simulink model "INTEGRATION_TEST_01"  (Simulink 8.1)
settings: Solver=ode4  StartTime=0.0  StopTime=inf  FixedStep=Ts  MaxStep=1e-3  RelTol=1e-3
PostLoadFcn:
  | INTEGRATION_TEST_01_init;
InitFcn:
  | INTEGRATION_TEST_01_init;
values from neighbouring files (symbols this model uses):
  Ts = 100E-6    (= 0.0001)    [INTEGRATION_TEST_01_init.m]
undefined symbols (not defined in the file or in its folder): cable_spec, fdesignblkfcn, gcbh, generic_ethernet_cb, Left, relay_par, type, V
libraries: powerlib_extras x14, rtio_opalrt_common x13, rtlab x10, cables_lib x6, breaker_lib x4, simulink_extras x4, simulink x4, Load_lib x3, rtio_generic_modbus x3, powerlib x2, ssn_lib x2, transformer_lib x2
(part 2 of 2)

== system INTEGRATION_TEST_01/SS_Relays_and_Woodward/HWCtrl/GR1 B AIN (CH00-15) ==
  AnalogIn : rtio_opalrt_common/AnalogIn  CtrlName='OpCtrl'  portNb=1  FcnNos=Slot 1 Module B Subsection 1  size=16  maxcount=8  count=8  numchan=8  sampleTime=0
      settings: AttributesFormatString=%<CtrlName>
  AnalogIn1 : rtio_opalrt_common/AnalogIn  CtrlName='OpCtrl'  portNb=2  FcnNos=Slot 1 Module B Subsection 2  size=16  maxcount=8  count=8  numchan=8  sampleTime=0
      settings: AttributesFormatString=%<CtrlName>
  Mux6 : Mux  Inputs=2
  Terminator2 : Terminator
  Terminator3 : Terminator
  Out1 : Outport
  wires:
  AnalogIn/1 -> Mux6/1
  AnalogIn1/1 -> Mux6/2
  AnalogIn/2 -> Terminator2/1
  AnalogIn1/2 -> Terminator3/1
  Mux6/1 -> Out1/1

== system INTEGRATION_TEST_01/SS_Relays_and_Woodward/HWCtrl/SEL751_DigitalAnalog_IO_OpBlocks ==
  note: This connector also services Genset #2 and  is
      | shared with Genset #1.  Use RJ45 connectors to
      |  intercept Genset #2 I/O (not used in this Device
      | Integration Test) and use for SEL-751
  note: Remove existing connections to Slot 3 I/O, if any
      | ans replace with connections shown below, or use
      | corresponding RJ45 connectors.  (Existing I/O, if any not
      |  used for this Device Integration Test)
  note: When the system uses the simulated
      | Secondary Controller the digital I/O
      | should be disabled.
  note: Copyright (c) 2016 Massachusetts Institute of Technology
      | Permission is hereby granted, free of charge, to any person obtaining a copy of this software and associated documentation files (the "Software"), to deal
      | in the Software without restriction, including without limitation the rights to use, copy, modify, merge, publish, distribute, sublicense, and/or sell copies of the
      | Software, and to permit persons to whom the Software is furnished to do so, subject to the following conditions:
      |
      | THE SOFTWARE IS PROVIDED "AS IS", WITHOUT WARRANTY OF ANY KIND, EXPRESS OR IMPLIED, INCLUDING BUT NOT LIMITED TO THE
      | WARRANTIES OF MERCHANTABILITY, FITNESS FOR A PARTICULAR PURPOSE AND NONINFRINGEMENT. IN NO EVENT SHALL THE AUTHORS
      | OR COPYRIGHT HOLDERS BE LIABLE FOR ANY CLAIM, DAMAGES OR OTHER LIABILITY, WHETHER IN AN ACTION OF CONTRACT, TORT OR
      | OTHERWISE, ARISING FROM, OUT OF OR IN CONNECTION WITH THE SOFTWARE OR THE USE OR OTHER DEALINGS IN THE SOFTWARE
  SEL751-01_ScaledSignals : Inport
  AnalogOut2 to SEL-751 : rtio_opalrt_common/AnalogOut  CtrlName='OpCtrl'  portNb=4  FcnNos=Slot 2 Module A Subsection 2  size=16  maxcount=8  count=8  numchan=8  israngeinput=off  voltagerange=[ -5 ... 5 ]  slot=1  side=0  mismatch=0  slotside=Slot_2_Module_A
      settings: AttributesFormatString=%<CtrlName>
  Bus Creator4 : BusCreator  Inputs=2
  Bus Selector4 : BusSelector  OutputSignals=To DigitalOut_to_SEL-751,To AnalogOut_to_SEL-751
  Data Type Conversion{,1..3} (4 alike) : DataTypeConversion
  Demux6 : Demux  Outputs=8
  DigitalIn from SEL-751 : rtio_opalrt_common/DigitalIn  CtrlName='OpCtrl'  portNb=6  FcnNos=Slot 3 Module A Subsection 2  size=1  maxcount=8  count=8  sampleTime=Ts  numchan=8
      settings: AttributesFormatString=%<CtrlName>
  DigitalOut to SEL-751 : rtio_opalrt_common/DigitalOut  CtrlName='OpCtrl'  portNb=6  FcnNos=Slot 3 Module B Subsection 2  size=1  maxcount=8  count=8  numchan=8
      settings: AttributesFormatString=%<CtrlName>
  S-R Flip-Flop : simulink_extras/Flip Flops/S-R Flip-Flop  initial_condition=1
  Terminator : Terminator
  Terminator1 : Terminator
  Terminator2 : Terminator
  SEL751-01_LogicTrip : Outport
  wires:
  DigitalOut to SEL-751/1 -> Terminator1/1
  AnalogOut2 to SEL-751/1 -> Terminator/1
  Demux6/2 -> Data Type Conversion1/1  "OUT102 Brkr reset"
  Demux6/1 -> Data Type Conversion/1  "OUT103 Brkr trip"
  Data Type Conversion3/1 -> Bus Creator4/2  "Logic_reset"
  Data Type Conversion/1 -> S-R Flip-Flop/1
  Bus Selector4/2 -> AnalogOut2 to SEL-751/1  "<To AnalogOut_to_SEL-751>"
  Bus Selector4/1 -> DigitalOut to SEL-751/1  "<To DigitalOut_to_SEL-751>"
  DigitalIn from SEL-751/2 -> Terminator2/1
  SEL751-01_ScaledSignals/1 -> Bus Selector4/1
  DigitalIn from SEL-751/1 -> Demux6/1
  Data Type Conversion1/1 -> S-R Flip-Flop/2
  Data Type Conversion2/1 -> Bus Creator4/1  "Logic_trip"
  Bus Creator4/1 -> SEL751-01_LogicTrip/1
  S-R Flip-Flop/1 -> Data Type Conversion2/1  "Logic_trip"
  S-R Flip-Flop/2 -> Data Type Conversion3/1  "Logic_reset"

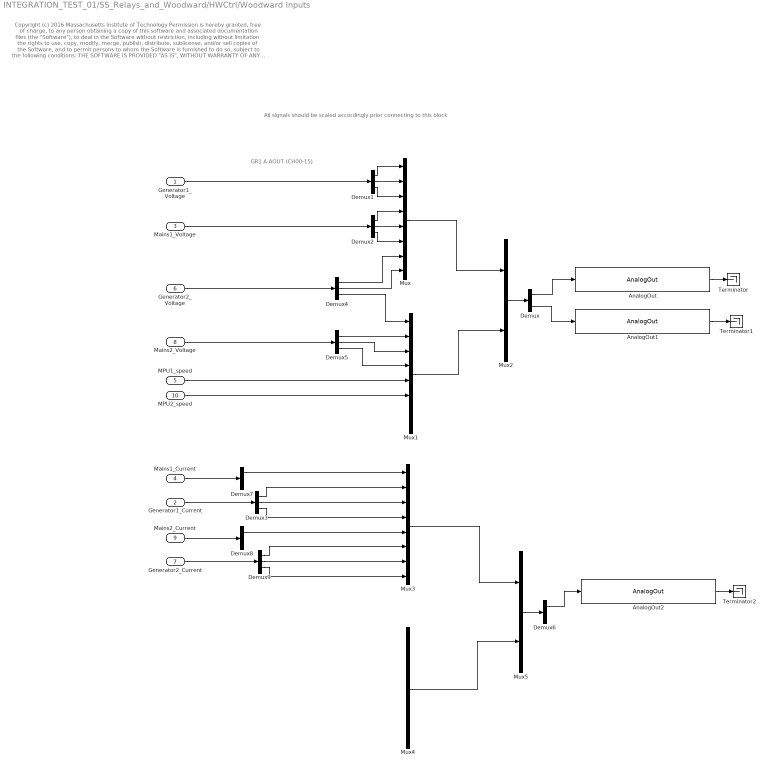
== system INTEGRATION_TEST_01/SS_Relays_and_Woodward/HWCtrl/Woodward Inputs ==
  note: All signals should be scaled accordingly prior connecting to this block
  note: GR1 A AOUT (CH00-15)
  note: Copyright (c) 2016 Massachusetts Institute of Technology
      | Permission is hereby granted, free of charge, to any person obtaining a copy of this software and associated documentation files (the "Software"), to deal
      | in the Software without restriction, including without limitation the rights to use, copy, modify, merge, publish, distribute, sublicense, and/or sell copies of the
      | Software, and to permit persons to whom the Software is furnished to do so, subject to the following conditions:
      |
      | THE SOFTWARE IS PROVIDED "AS IS", WITHOUT WARRANTY OF ANY KIND, EXPRESS OR IMPLIED, INCLUDING BUT NOT LIMITED TO THE
      | WARRANTIES OF MERCHANTABILITY, FITNESS FOR A PARTICULAR PURPOSE AND NONINFRINGEMENT. IN NO EVENT SHALL THE AUTHORS
      | OR COPYRIGHT HOLDERS BE LIABLE FOR ANY CLAIM, DAMAGES OR OTHER LIABILITY, WHETHER IN AN ACTION OF CONTRACT, TORT OR
      | OTHERWISE, ARISING FROM, OUT OF OR IN CONNECTION WITH THE SOFTWARE OR THE USE OR OTHER DEALINGS IN THE SOFTWARE
  Generator1_Voltage : Inport
  Generator1_Current : Inport  Port=2
  Mains1_Voltage : Inport  Port=3
  Mains1_Current : Inport  Port=4
  MPU1_speed : Inport  Port=5
  Generator2_Voltage : Inport  Port=6
  Generator2_Current : Inport  Port=7
  Mains2_Voltage : Inport  Port=8
  Mains2_Current : Inport  Port=9
  MPU2_speed : Inport  Port=10
  AnalogOut : rtio_opalrt_common/AnalogOut  CtrlName='OpCtrl'  portNb=1  FcnNos=Slot 1 Module A Subsection 1  size=16  maxcount=8  count=8  numchan=8  israngeinput=off  voltagerange=[-16 ... 16]  slot=0  side=0  mismatch=0  slotside=Slot_1_Module_A
      settings: AttributesFormatString=%<CtrlName>
  AnalogOut1 : rtio_opalrt_common/AnalogOut  CtrlName='OpCtrl'  portNb=2  FcnNos=Slot 1 Module A Subsection 2  size=16  maxcount=8  count=8  numchan=8  israngeinput=off  voltagerange=[-16 ... 16]  slot=0  side=0  mismatch=0  slotside=Slot_1_Module_A
      settings: AttributesFormatString=%<CtrlName>
  AnalogOut2 : rtio_opalrt_common/AnalogOut  CtrlName='OpCtrl'  portNb=3  FcnNos=Slot 2 Module A Subsection 1  size=16  maxcount=8  count=8  numchan=8  israngeinput=off  voltagerange=[-16 ... 16]  slot=1  side=0  mismatch=0  slotside=Slot_2_Module_A
      settings: AttributesFormatString=%<CtrlName>
  Demux : Demux  Outputs=2
  Demux{1..5,7..9} (8 alike) : Demux  Outputs=3
  Demux6 : Demux  Outputs=2
  Mux{,1,3..4} (4 alike) : Mux  Inputs=8
  Mux2 : Mux  Inputs=2
  Mux5 : Mux  Inputs=2
  Terminator : Terminator
  Terminator1 : Terminator
  Terminator2 : Terminator
  wires:
  Demux9/3 -> Mux3/8
  Demux9/2 -> Mux3/7
  Demux9/1 -> Mux3/6
  Generator2_Current/1 -> Demux9/1
  Demux8/1 -> Mux3/5
  Mains2_Current/1 -> Demux8/1
  MPU2_speed/1 -> Mux1/6
  Generator2_Voltage/1 -> Demux4/1
  Mains2_Voltage/1 -> Demux5/1
  Demux7/1 -> Mux3/1
  Mains1_Current/1 -> Demux7/1
  Demux3/3 -> Mux3/4
  Demux3/2 -> Mux3/3
  Demux3/1 -> Mux3/2
  Generator1_Current/1 -> Demux3/1
  AnalogOut2/1 -> Terminator2/1
  Demux6/1 -> AnalogOut2/1
  Mux3/1 -> Mux5/1
  Mux4/1 -> Mux5/2
  Mux5/1 -> Demux6/1
  Demux5/3 -> Mux1/4
  Demux5/2 -> Mux1/3
  Demux5/1 -> Mux1/2
  Demux4/3 -> Mux1/1
  Demux4/2 -> Mux/8
  Demux4/1 -> Mux/7
  MPU1_speed/1 -> Mux1/5
  Demux2/3 -> Mux/6
  Demux2/2 -> Mux/5
  Demux2/1 -> Mux/4
  Demux1/3 -> Mux/3
  Demux1/2 -> Mux/2
  Demux1/1 -> Mux/1
  AnalogOut/1 -> Terminator/1
  AnalogOut1/1 -> Terminator1/1
  Demux/1 -> AnalogOut/1
  Demux/2 -> AnalogOut1/1
  Mux/1 -> Mux2/1
  Mux1/1 -> Mux2/2
  Mux2/1 -> Demux/1
  Generator1_Voltage/1 -> Demux1/1
  Mains1_Voltage/1 -> Demux2/1

== system INTEGRATION_TEST_01/SS_Relays_and_Woodward/HWCtrl/Woodward Outputs - NGCHP - Gen1 ==
  note: Copyright (c) 2016 Massachusetts Institute of Technology
      | Permission is hereby granted, free of charge, to any person obtaining a copy of this software and associated documentation files (the "Software"), to deal
      | in the Software without restriction, including without limitation the rights to use, copy, modify, merge, publish, distribute, sublicense, and/or sell copies of the
      | Software, and to permit persons to whom the Software is furnished to do so, subject to the following conditions:
      |
      | THE SOFTWARE IS PROVIDED "AS IS", WITHOUT WARRANTY OF ANY KIND, EXPRESS OR IMPLIED, INCLUDING BUT NOT LIMITED TO THE
      | WARRANTIES OF MERCHANTABILITY, FITNESS FOR A PARTICULAR PURPOSE AND NONINFRINGEMENT. IN NO EVENT SHALL THE AUTHORS
      | OR COPYRIGHT HOLDERS BE LIABLE FOR ANY CLAIM, DAMAGES OR OTHER LIABILITY, WHETHER IN AN ACTION OF CONTRACT, TORT OR
      | OTHERWISE, ARISING FROM, OUT OF OR IN CONNECTION WITH THE SOFTWARE OR THE USE OR OTHER DEALINGS IN THE SOFTWARE
  Gen1 MCB Status : Inport
  WoodwardBias : Inport  Port=2
  Bus Creator1 : BusCreator  Inputs=1
  DIO - Gr3 : Subsystem
  DIO - Woodward : Subsystem
  DOUT type config : Subsystem
  Woodward Primary Inputs - Gen1 : Subsystem
  Digital Inputs : Outport
  Gen1 Gov and AVR : Outport  Port=2
  Gen1 Fuel Enable : Outport  Port=3
  Gen1 GCB : Outport  Port=4
  Gen1 MCB : Outport  Port=5
  wires:
  Gen1 MCB Status/1 -> DIO - Woodward/2(Gen1 MCB Status)
  DIO - Woodward/1(Gen1 Fuel Enable) -> Gen1 Fuel Enable/1
  DIO - Woodward/3(Gen1 MCB) -> Gen1 MCB/1
  DIO - Woodward/2(Gen1 GCB) -> Gen1 GCB/1
  WoodwardBias/1 -> Woodward Primary Inputs - Gen1/1(WoodwardBias)
  Woodward Primary Inputs - Gen1/1(Gen1 Gov and AVR) -> Gen1 Gov and AVR/1
  Bus Creator1/1 -> Digital Inputs/1
  DIO - Gr3/1(DIn) -> Bus Creator1/1, DIO - Woodward/1(Din_Wood)  "DIN"
  DIO - Woodward/4(DIn1) -> DIO - Gr3/1(Dout)

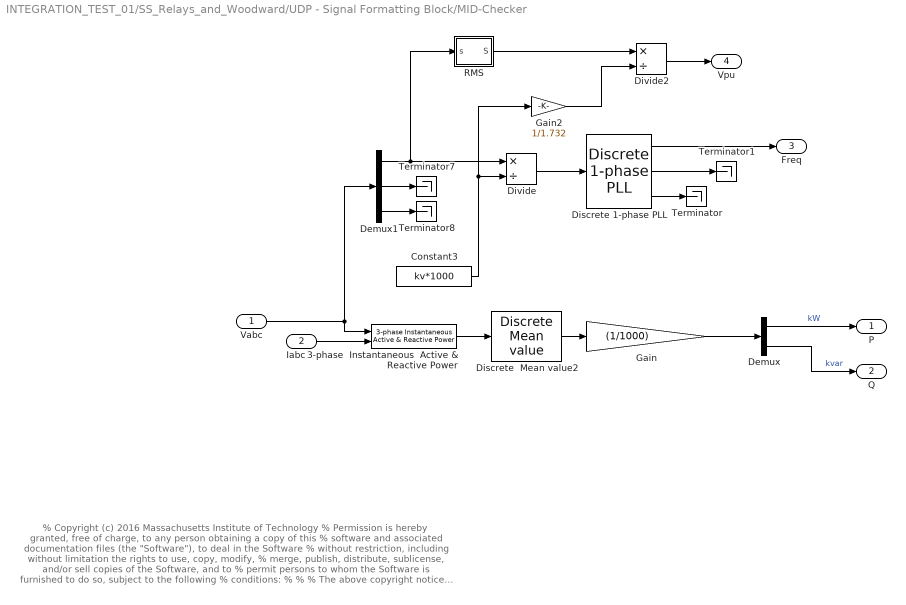
== system INTEGRATION_TEST_01/SS_Relays_and_Woodward/UDP - Signal Formatting Block/MID-Checker ==
  note: % Copyright (c) 2016 Massachusetts Institute of Technology
      | % Permission is hereby granted, free of charge, to any person obtaining a copy of this
      | % software and associated documentation files (the "Software"), to deal in the Software
      | % without restriction, including without limitation the rights to use, copy, modify,
      | % merge, publish, distribute, sublicense, and/or sell copies of the Software, and to
      | % permit persons to whom the Software is furnished to do so, subject to the following
      | % conditions:
      | %
      | %
      | % The above copyright notice and this permission notice shall be included in
      | % all copies or substantial portions of the Software.
      | %
      | % THE SOFTWARE IS PROVIDED "AS IS", WITHOUT WARRANTY OF ANY KIND, EXPRESS OR IMPLIED,
      | % INCLUDING BUT NOT LIMITED TO THE WARRANTIES OF MERCHANTABILITY, FITNESS FOR A
      | % PARTICULAR PURPOSE AND NONINFRINGEMENT. IN NO EVENT SHALL THE AUTHORS OR COPYRIGHT
      | % HOLDERS BE LIABLE FOR ANY CLAIM, DAMAGES OR OTHER LIABILITY, WHETHER IN AN ACTION
      | % OF CONTRACT, TORT OR OTHERWISE, ARISING FROM, OUT OF OR IN CONNECTION WITH THE
      | % SOFTWARE OR THE USE OR OTHER DEALINGS IN THE SOFTWARE.
      | %
      | %
      | %%
  Vabc : Inport
  Iabc : Inport  Port=2
  3-phase  Instantaneous  Active & Reactive Power : powerlib_extras/Measurements/3-phase  Instantaneous  Active & Reactive Power
  Constant3 : Constant  Value=kv*1000
  Demux : Demux  Outputs=2
  Demux1 : Demux  Outputs=3
  Discrete 1-phase PLL : powerlib_extras/Discrete  Control Blocks/Discrete 1-phase PLL  Fmin=45  Par_Init=[0 60]  ParK=[ 180 3200 1]  Ts=Ts  AGC=on
  Discrete  Mean value2 : powerlib_extras/Discrete Measurements/Discrete  Mean value  Freq=60  Vinit=0  Ts=Ts
  Divide : Product  Inputs=*/
  Divide2 : Product  Inputs=*/
  Gain : Gain  Gain=(1/1000)
  Gain2 : Gain  Gain=1/1.732
  RMS : Subsystem
  Terminator{,1,7..8} (4 alike) : Terminator
  P : Outport
  Q : Outport  Port=2
  Freq : Outport  Port=3
  Vpu : Outport  Port=4
  wires:
  Demux/2 -> Q/1  "kvar"
  Demux/1 -> P/1  "kW"
  Iabc/1 -> 3-phase  Instantaneous  Active & Reactive Power/2
  Discrete  Mean value2/1 -> Gain/1
  3-phase  Instantaneous  Active & Reactive Power/1 -> Discrete  Mean value2/1
  Gain/1 -> Demux/1
  Discrete 1-phase PLL/1 -> Freq/1
  Discrete 1-phase PLL/3 -> Terminator/1
  Divide/1 -> Discrete 1-phase PLL/1
  Discrete 1-phase PLL/2 -> Terminator1/1
  Demux1/1 -> RMS/1(s), Divide/1
  Demux1/2 -> Terminator7/1
  Demux1/3 -> Terminator8/1
  Vabc/1 -> 3-phase  Instantaneous  Active & Reactive Power/1, Demux1/1
  Constant3/1 -> Divide/2, Gain2/1
  Gain2/1 -> Divide2/2
  RMS/1(S) -> Divide2/1
  Divide2/1 -> Vpu/1

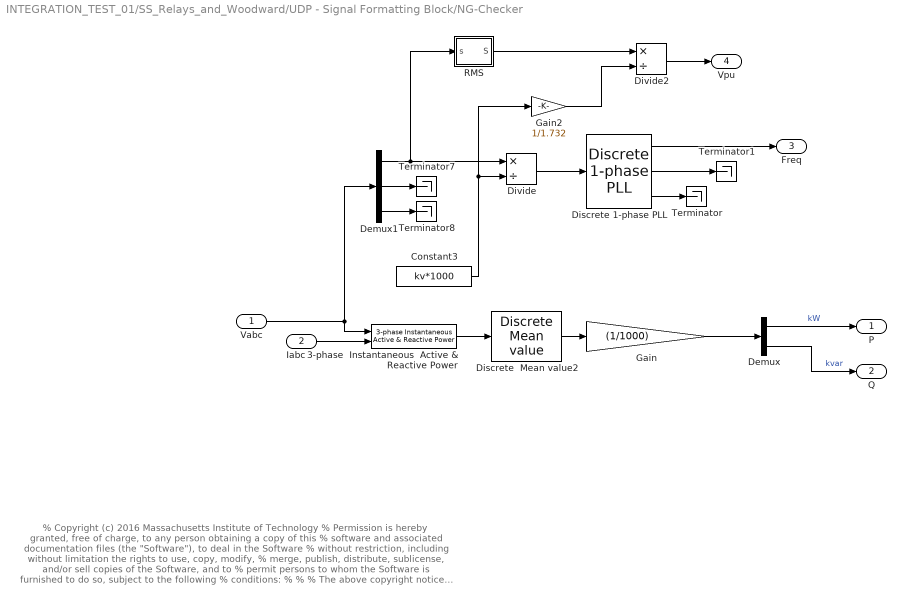
== system INTEGRATION_TEST_01/SS_Relays_and_Woodward/UDP - Signal Formatting Block/NG-Checker ==
  note: % Copyright (c) 2016 Massachusetts Institute of Technology
      | % Permission is hereby granted, free of charge, to any person obtaining a copy of this
      | % software and associated documentation files (the "Software"), to deal in the Software
      | % without restriction, including without limitation the rights to use, copy, modify,
      | % merge, publish, distribute, sublicense, and/or sell copies of the Software, and to
      | % permit persons to whom the Software is furnished to do so, subject to the following
      | % conditions:
      | %
      | %
      | % The above copyright notice and this permission notice shall be included in
      | % all copies or substantial portions of the Software.
      | %
      | % THE SOFTWARE IS PROVIDED "AS IS", WITHOUT WARRANTY OF ANY KIND, EXPRESS OR IMPLIED,
      | % INCLUDING BUT NOT LIMITED TO THE WARRANTIES OF MERCHANTABILITY, FITNESS FOR A
      | % PARTICULAR PURPOSE AND NONINFRINGEMENT. IN NO EVENT SHALL THE AUTHORS OR COPYRIGHT
      | % HOLDERS BE LIABLE FOR ANY CLAIM, DAMAGES OR OTHER LIABILITY, WHETHER IN AN ACTION
      | % OF CONTRACT, TORT OR OTHERWISE, ARISING FROM, OUT OF OR IN CONNECTION WITH THE
      | % SOFTWARE OR THE USE OR OTHER DEALINGS IN THE SOFTWARE.
      | %
      | %
      | %%
  Vabc : Inport
  Iabc : Inport  Port=2
  3-phase  Instantaneous  Active & Reactive Power : powerlib_extras/Measurements/3-phase  Instantaneous  Active & Reactive Power
  Constant3 : Constant  Value=kv*1000
  Demux : Demux  Outputs=2
  Demux1 : Demux  Outputs=3
  Discrete 1-phase PLL : powerlib_extras/Discrete  Control Blocks/Discrete 1-phase PLL  Fmin=45  Par_Init=[0 60]  ParK=[ 180 3200 1]  Ts=Ts  AGC=on
  Discrete  Mean value2 : powerlib_extras/Discrete Measurements/Discrete  Mean value  Freq=60  Vinit=0  Ts=Ts
  Divide : Product  Inputs=*/
  Divide2 : Product  Inputs=*/
  Gain : Gain  Gain=(1/1000)
  Gain2 : Gain  Gain=1/1.732
  RMS : Subsystem
  Terminator{,1,7..8} (4 alike) : Terminator
  P : Outport
  Q : Outport  Port=2
  Freq : Outport  Port=3
  Vpu : Outport  Port=4
  wires:
  Demux/2 -> Q/1  "kvar"
  Demux/1 -> P/1  "kW"
  Iabc/1 -> 3-phase  Instantaneous  Active & Reactive Power/2
  Discrete  Mean value2/1 -> Gain/1
  3-phase  Instantaneous  Active & Reactive Power/1 -> Discrete  Mean value2/1
  Gain/1 -> Demux/1
  Discrete 1-phase PLL/1 -> Freq/1
  Discrete 1-phase PLL/3 -> Terminator/1
  Divide/1 -> Discrete 1-phase PLL/1
  Discrete 1-phase PLL/2 -> Terminator1/1
  Demux1/1 -> RMS/1(s), Divide/1
  Demux1/2 -> Terminator7/1
  Demux1/3 -> Terminator8/1
  Vabc/1 -> 3-phase  Instantaneous  Active & Reactive Power/1, Demux1/1
  Constant3/1 -> Divide/2, Gain2/1
  Gain2/1 -> Divide2/2
  RMS/1(S) -> Divide2/1
  Divide2/1 -> Vpu/1

== system INTEGRATION_TEST_01/SS_Relays_and_Woodward/UDP - Signal Formatting Block/RMS ==
  s : Inport
  Discrete  Mean value6 : powerlib_extras/Discrete Measurements/Discrete  Mean value  Freq=60  Vinit=0  Ts=Ts
  Product3 : Product  RndMeth=Zero
  Signed Sqrt : Sqrt  SaturateOnIntegerOverflow=on
  S : Outport
  wires:
  Signed Sqrt/1 -> S/1
  Discrete  Mean value6/1 -> Signed Sqrt/1
  Product3/1 -> Discrete  Mean value6/1
  s/1 -> Product3/2, Product3/1

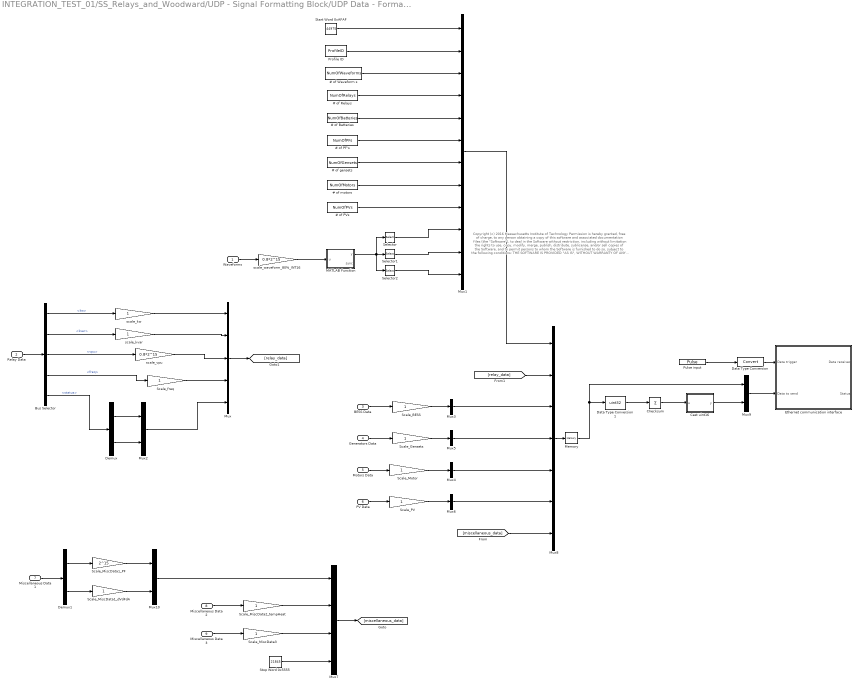
== system INTEGRATION_TEST_01/SS_Relays_and_Woodward/UDP - Signal Formatting Block/UDP Data - Formatted Send - Integartion Test 1 ==
  note: Copyright (c) 2016 Massachusetts Institute of Technology
      | Permission is hereby granted, free of charge, to any person obtaining a copy of this software and associated documentation files (the "Software"), to deal
      | in the Software without restriction, including without limitation the rights to use, copy, modify, merge, publish, distribute, sublicense, and/or sell copies of the
      | Software, and to permit persons to whom the Software is furnished to do so, subject to the following conditions:
      |
      | THE SOFTWARE IS PROVIDED "AS IS", WITHOUT WARRANTY OF ANY KIND, EXPRESS OR IMPLIED, INCLUDING BUT NOT LIMITED TO THE
      | WARRANTIES OF MERCHANTABILITY, FITNESS FOR A PARTICULAR PURPOSE AND NONINFRINGEMENT. IN NO EVENT SHALL THE AUTHORS
      | OR COPYRIGHT HOLDERS BE LIABLE FOR ANY CLAIM, DAMAGES OR OTHER LIABILITY, WHETHER IN AN ACTION OF CONTRACT, TORT OR
      | OTHERWISE, ARISING FROM, OUT OF OR IN CONNECTION WITH THE SOFTWARE OR THE USE OR OTHER DEALINGS IN THE SOFTWARE
  Waveforms : Inport  PortDimensions=3
  Relay Data : Inport  Port=2
  BESS Data : Inport  Port=3
  Generators Data : Inport  Port=4
  Motors Data : Inport  Port=5
  PV Data : Inport  Port=6
  Miscellaneous Data 1 : Inport  Port=7
  Miscellaneous Data 2 : Inport  Port=8
  Miscellaneous Data 3 : Inport  Port=9
  " # of motors" : Constant  Value=NumOfMotors  OutDataTypeStr=double
  # of Batteries : Constant  Value=NumOfBatteries  OutDataTypeStr=double
  # of PF's : Constant  Value=NumOfPFs  OutDataTypeStr=double
  # of PVs : Constant  Value=NumOfPVs  OutDataTypeStr=double
  # of Relays : Constant  Value=NumOfRelays  OutDataTypeStr=double
  # of Waveform s : Constant  Value=NumOfWaveforms  OutDataTypeStr=double
  # of gensets : Constant  Value=NumOfGensets  OutDataTypeStr=double
  Bus Selector : BusSelector  OutputSignals=kw,kvar,vpu,freq,status
  Cast uint16 : MATLAB Function  TreatAsAtomicUnit=on
  Checksum : Sum  Inputs=+
  Data Type Conversion : DataTypeConversion
  Data Type Conversion1 : DataTypeConversion  OutDataTypeStr=uint32  ConvertRealWorld=Stored Integer (SI)  RndMeth=Nearest
  Demux : Demux  Outputs=[2 2]
  Demux1 : Demux  Outputs=[1 3]
  Ethernet communication interface : Subsystem  mask(AsyncEthernet){ctrl_id=1, nbr_to_remote_endpoint=730, type_to_remote_endpoint=INT16, offset_to_remote_endpoint=0, swap_tx=off, nbr_from_remote_endpoint=4, type_from_remote_endpoint=UINT16, offset_from_remote_endpoint=0, swap_rx=off, exe_name='AsyncEthernet', nic_name='eth0', protocol=UDP, tcp_mode=Server, port=7200, remote_ip='255.255.255.255'}
      mask prompts: ctrl_id "Controller ID"; nbr_to_remote_endpoint "Number of data to send"; type_to_remote_endpoint "Type of data to send"; offset_to_remote_endpoint "Byte offset of transmission buffer"; swap_tx "Swap data endianness before transmission"; nbr_from_remote_endpoint "Number of data expected to be received"; type_from_remote_endpoint "Type of data expected to be received"; offset_from_remote_endpoint "Byte offset of reception buffer"; swap_rx "Swap data endianness after reception"; exe_name "Executable name"; nic_name "Network interface name"; tcp_mode "TCP mode"; port "Port number"; remote_ip "Remote IP address"
      mask help: This block is used as a communication interface to send data to a remote dedevice and receive data from it.
      mask Help: eval('rtlab_io_help(''Generic/Ethernet/Ethernet_interface.htm'');');
      mask Callback ctrl_id:
      | var = get_param(gcb,'ctrl_id');
      | set_param([gcb '/AsyncEthernetCtrl'],'ctrl_id',var)
      mask Callback nbr_to_remote_endpoint:
      | var = get_param(gcb,'nbr_to_remote_endpoint');
      | set_param([gcb '/AsyncEthernetCtrl'],'nbr_to_remote_endpoint',var)
      mask TypeOptions type_to_remote_endpoint: UINT8 | INT8 | UINT16 | INT16 | UINT32 | INT32 | FLOAT | DOUBLE
      mask Callback type_to_remote_endpoint:
      | var = get_param(gcb,'type_to_remote_endpoint');
      | set_param([gcb '/AsyncEthernetCtrl'],'type_to_remote_endpoint',var)
      mask Callback offset_to_remote_endpoint:
      | var = get_param(gcb,'offset_to_remote_endpoint');
      | set_param([gcb '/AsyncEthernetCtrl'],'offset_to_remote_endpoint',var)
      mask Callback swap_tx:
      | var = get_param(gcb,'swap_tx');
      | set_param([gcb '/AsyncEthernetCtrl'],'swap_tx',var)
      mask Callback nbr_from_remote_endpoint:
      | var = get_param(gcb,'nbr_from_remote_endpoint');
      | set_param([gcb '/AsyncEthernetCtrl'],'nbr_from_remote_endpoint',var)
      mask TypeOptions type_from_remote_endpoint: UINT8 | INT8 | UINT16 | INT16 | UINT32 | INT32 | FLOAT | DOUBLE
      mask Callback type_from_remote_endpoint:
      | var = get_param(gcb,'type_from_remote_endpoint');
      | set_param([gcb '/AsyncEthernetCtrl'],'type_from_remote_endpoint',var)
      mask Callback offset_from_remote_endpoint:
      | var = get_param(gcb,'offset_from_remote_endpoint');
      | set_param([gcb '/AsyncEthernetCtrl'],'offset_from_remote_endpoint',var)
      mask Callback swap_rx:
      | var = get_param(gcb,'swap_rx');
      | set_param([gcb '/AsyncEthernetCtrl'],'swap_rx',var)
      mask Callback exe_name:
      | str = get_param(gcb,'exe_name');
      | 
      | if exist('str','var')
      |     str = eval(str);
      | end
      | 
      | set_param([gcb '/AsyncEthernetCtrl'],'exe_name',str)
      mask Callback nic_name:
      | str = get_param(gcb,'nic_name');
      | 
      | if exist('str','var')
      |     str = eval(str);
      | end
      | 
      | set_param([gcb '/AsyncEthernetCtrl'],'nic_name',str)
      mask TypeOptions protocol: UDP | TCP
      mask Callback protocol: generic_ethernet_cb('protocol')
      mask TypeOptions tcp_mode: Client | Server
      mask Callback tcp_mode: generic_ethernet_cb('tcp_mode')
      mask Callback port:
      | var = get_param(gcb,'port');
      | set_param([gcb '/AsyncEthernetCtrl'],'port',var)
      mask Callback remote_ip:
      | str = get_param(gcb,'remote_ip');
      | 
      | if exist('str','var')
      |     str = eval(str);
      | end
      | 
      | set_param([gcb '/AsyncEthernetCtrl'],'remote_ip',str)
  MATLAB Function : MATLAB Function  TreatAsAtomicUnit=on
  Memory : Memory
  Mux : Mux  Inputs=5
  Mux1 : Mux  Inputs=12
  Mux10 : Mux  Inputs=2
  Mux2 : Mux  Inputs=2
  Mux{3..6} (4 alike) : Mux  Inputs=1
  Mux7 : Mux
  Mux8 : Mux  Inputs=7
  Mux9 : Mux  Inputs=2
  Profile ID : Constant  Value=ProfileID  OutDataTypeStr=double
  Pulse input : DiscretePulseGenerator  PulseType=Time based  Period=1/5
  Scale_BESS : Gain
  Scale_Gensets : Gain
  Scale_MiscData1_PF : Gain  Gain=2^15
  Scale_MiscData1_dVdFdA : Gain
  Scale_MiscData2_tempHeat : Gain
  Scale_MiscData3 : Gain
  Scale_Motor : Gain
  Scale_PV : Gain
  Scale_freq : Gain
  Selector : Selector  NumberOfDimensions=2  InputPortWidth=3  IndexOptions=Index vector (dialog),Select all  Indices=[1],1  OutputSizes=208,1
  Selector1 : Selector  NumberOfDimensions=2  InputPortWidth=3  IndexOptions=Index vector (dialog),Select all  Indices=[2],1  OutputSizes=208,1
  Selector2 : Selector  NumberOfDimensions=2  InputPortWidth=3  IndexOptions=Index vector (dialog),Select all  Indices=[3],1  OutputSizes=208,1
  Start Word 0xAFAF : Constant  Value=44975  OutDataTypeStr=double
  Stop Word 0x5555 : Constant  Value=21845  OutDataTypeStr=double
  scale_kvar : Gain
  scale_kw : Gain
  scale_vpu : Gain  Gain=0.8*2^15
  scale_waveform_80%_INT16 : Gain  Gain=0.8*2^15
  wires:
  # of Waveform s/1 -> Mux1/3
  Profile ID/1 -> Mux1/2
  Start Word 0xAFAF/1 -> Mux1/1
  Pulse input/1 -> Data Type Conversion/1
  Data Type Conversion/1 -> Ethernet communication interface/1(Data trigger)
  Waveforms/1 -> scale_waveform_80%_INT16/1
  MATLAB Function/1(y) -> Selector/1, Selector1/1, Selector2/1
  Mux1/1 -> Mux8/1
  Mux8/1 -> Memory/1
  Checksum/1 -> Cast uint16/1(u)
  Cast uint16/1(y) -> Mux9/2
  Mux9/1 -> Ethernet communication interface/2(Data to send)
  Bus Selector/5 -> Demux/1  "<status>"
  Data Type Conversion1/1 -> Checksum/1
  scale_waveform_80%_INT16/1 -> MATLAB Function/1(u)
  Stop Word 0x5555/1 -> Mux7/4
  Miscellaneous Data 2/1 -> Scale_MiscData2_tempHeat/1
  Demux/1 -> Mux2/1
  Demux/2 -> Mux2/2
  # of PVs/1 -> Mux1/9
  " # of motors"/1 -> Mux1/8
  # of gensets/1 -> Mux1/7
  # of PF's/1 -> Mux1/6
  # of Batteries/1 -> Mux1/5
  # of Relays/1 -> Mux1/4
  Selector1/1 -> Mux1/11
  Selector2/1 -> Mux1/12
  Selector/1 -> Mux1/10
  Relay Data/1 -> Bus Selector/1
  Bus Selector/3 -> scale_vpu/1  "<vpu>"
  Miscellaneous Data 3/1 -> Scale_MiscData3/1
  Bus Selector/1 -> scale_kw/1  "<kw>"
  Bus Selector/2 -> scale_kvar/1  "<kvar>"
  scale_vpu/1 -> Mux/3
  Bus Selector/4 -> Scale_freq/1  "<freq>"
  Mux2/1 -> Mux/5
  BESS Data/1 -> Scale_BESS/1
  Motors Data/1 -> Scale_Motor/1
  Generators Data/1 -> Scale_Gensets/1
  PV Data/1 -> Scale_PV/1
  [miscellaneous_data] -> Mux8/7
  Mux7/1 -> [miscellaneous_data]
  [relay_data] -> Mux8/2
  Mux/1 -> [relay_data]
  Mux3/1 -> Mux8/3
  Mux5/1 -> Mux8/4
  Mux4/1 -> Mux8/5
  Mux6/1 -> Mux8/6
  Miscellaneous Data 1/1 -> Demux1/1
  Demux1/1 -> Scale_MiscData1_PF/1
  Scale_MiscData1_PF/1 -> Mux10/1
  Demux1/2 -> Scale_MiscData1_dVdFdA/1
  Mux10/1 -> Mux7/1
  scale_kw/1 -> Mux/1
  scale_kvar/1 -> Mux/2
  Scale_freq/1 -> Mux/4
  Scale_BESS/1 -> Mux3/1
  Scale_Gensets/1 -> Mux5/1
  Scale_Motor/1 -> Mux4/1
  Scale_PV/1 -> Mux6/1
  Scale_MiscData3/1 -> Mux7/3
  Scale_MiscData2_tempHeat/1 -> Mux7/2
  Scale_MiscData1_dVdFdA/1 -> Mux10/2
  Memory/1 -> Mux9/1, Data Type Conversion1/1

== system INTEGRATION_TEST_01/SS_Relays_and_Woodward/UDP - Signal Formatting Block/set of 1ph PLLs ==
  V_bus : Inport
  V_line : Inport  Port=2
  VRMSLL : Inport  Port=3
  Discrete 1-phase PLL : powerlib_extras/Discrete  Control Blocks/Discrete 1-phase PLL  Fmin=45  Par_Init=[0 60]  ParK=[ 180 3200 1]  Ts=Ts  AGC=on
  Discrete 1-phase PLL1 : powerlib_extras/Discrete  Control Blocks/Discrete 1-phase PLL  Fmin=45  Par_Init=[0 60]  ParK=[ 180 3200 1]  Ts=Ts  AGC=on
  Divide : Product  Inputs=*/
  Divide1 : Product  Inputs=*/
  Terminator : Terminator
  Terminator1 : Terminator
  f_bus : Outport
  f_line : Outport  Port=2
  wt_bus : Outport  Port=3
  wt_line : Outport  Port=4
  wires:
  V_bus/1 -> Divide1/1
  Divide1/1 -> Discrete 1-phase PLL1/1
  V_line/1 -> Divide/1
  Divide/1 -> Discrete 1-phase PLL/1
  VRMSLL/1 -> Divide1/2, Divide/2
  Discrete 1-phase PLL1/1 -> f_bus/1
  Discrete 1-phase PLL1/2 -> wt_bus/1
  Discrete 1-phase PLL/1 -> f_line/1
  Discrete 1-phase PLL/2 -> wt_line/1
  Discrete 1-phase PLL/3 -> Terminator/1
  Discrete 1-phase PLL1/3 -> Terminator1/1

== system INTEGRATION_TEST_01/SS_Relays_and_Woodward/HWCtrl/Woodward Outputs - NGCHP - Gen1/DIO - Gr3 ==
  Dout : Inport
  Bus Creator : BusCreator  Inputs=1
  Bus Selector : BusSelector  OutputSignals=DI_CH00-07  OutputAsBus=on
  Conditioning : Subsystem
  DigitalIn : rtio_opalrt_common/DigitalIn  CtrlName='OpCtrl'  portNb=5  FcnNos=Slot 3 Module A Subsection 1  size=1  maxcount=8  count=8  sampleTime=0  numchan=8
      settings: AttributesFormatString=%<CtrlName>
  DigitalOut : rtio_opalrt_common/DigitalOut  CtrlName='OpCtrl'  portNb=5  FcnNos=Slot 3 Module B Subsection 1  size=1  maxcount=8  count=8  numchan=8
      settings: AttributesFormatString=%<CtrlName>
  Terminator3 : Terminator
  Terminator5 : Terminator
  DIn : Outport
  wires:
  Conditioning/1(Out1) -> Bus Creator/1
  Bus Creator/1 -> DIn/1
  DigitalIn/1 -> Conditioning/1(In1)  "DI_CH00-07"
  DigitalIn/2 -> Terminator5/1
  Bus Selector/1 -> DigitalOut/1
  Dout/1 -> Bus Selector/1
  DigitalOut/1 -> Terminator3/1

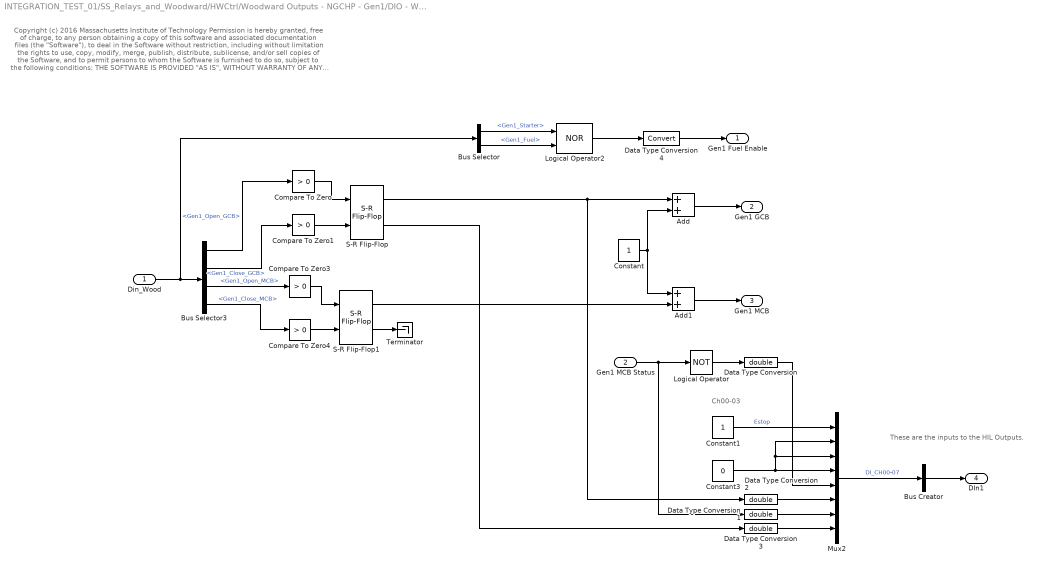
== system INTEGRATION_TEST_01/SS_Relays_and_Woodward/HWCtrl/Woodward Outputs - NGCHP - Gen1/DIO - Woodward ==
  note: Copyright (c) 2016 Massachusetts Institute of Technology
      | Permission is hereby granted, free of charge, to any person obtaining a copy of this software and associated documentation files (the "Software"), to deal
      | in the Software without restriction, including without limitation the rights to use, copy, modify, merge, publish, distribute, sublicense, and/or sell copies of the
      | Software, and to permit persons to whom the Software is furnished to do so, subject to the following conditions:
      |
      | THE SOFTWARE IS PROVIDED "AS IS", WITHOUT WARRANTY OF ANY KIND, EXPRESS OR IMPLIED, INCLUDING BUT NOT LIMITED TO THE
      | WARRANTIES OF MERCHANTABILITY, FITNESS FOR A PARTICULAR PURPOSE AND NONINFRINGEMENT. IN NO EVENT SHALL THE AUTHORS
      | OR COPYRIGHT HOLDERS BE LIABLE FOR ANY CLAIM, DAMAGES OR OTHER LIABILITY, WHETHER IN AN ACTION OF CONTRACT, TORT OR
      | OTHERWISE, ARISING FROM, OUT OF OR IN CONNECTION WITH THE SOFTWARE OR THE USE OR OTHER DEALINGS IN THE SOFTWARE
  note: Ch00-03
  note: These are the inputs to
      | the HIL Outputs.
  Din_Wood : Inport
  Gen1 MCB Status : Inport  Port=2
  Add : Sum
  Add1 : Sum
  Bus Creator : BusCreator  Inputs=1
  Bus Selector : BusSelector  OutputSignals=DI_CH00-07.Gen1_Starter,DI_CH00-07.Gen1_Fuel
  Bus Selector3 : BusSelector  OutputSignals=DI_CH00-07.Gen1_Open_GCB,DI_CH00-07.Gen1_Close_GCB,DI_CH00-07.Gen1_Open_MCB,DI_CH00-07.Gen1_Close_MCB
  Compare To Zero{,1,3..4} (4 alike) : simulink/Logic and Bit Operations/Compare To Zero  relop=>  OutDataTypeStr=boolean
  Constant : Constant
  Constant1 : Constant
  Constant3 : Constant  Value=0
  Data Type Conversion{,1..3} (4 alike) : DataTypeConversion  OutDataTypeStr=double
  Data Type Conversion4 : DataTypeConversion
  Logical Operator : Logic  Operator=NOT  AllPortsSameDT=off  OutDataTypeStr=boolean
  Logical Operator2 : Logic  Operator=NOR  AllPortsSameDT=off  OutDataTypeStr=boolean
  Mux2 : Mux  Inputs=8
  S-R Flip-Flop : simulink_extras/Flip Flops/S-R Flip-Flop  initial_condition=1
  S-R Flip-Flop1 : simulink_extras/Flip Flops/S-R Flip-Flop  initial_condition=1
  Terminator : Terminator
  Gen1 Fuel Enable : Outport
  Gen1 GCB : Outport  Port=2
  Gen1 MCB : Outport  Port=3
  DIn1 : Outport  Port=4
  wires:
  S-R Flip-Flop1/2 -> Terminator/1
  Data Type Conversion2/1 -> Mux2/6
  Data Type Conversion1/1 -> Mux2/7
  Data Type Conversion3/1 -> Mux2/8
  Mux2/1 -> Bus Creator/1  "DI_CH00-07"
  Constant3/1 -> Mux2/2, Mux2/3, Mux2/4
  Logical Operator2/1 -> Data Type Conversion4/1
  Logical Operator/1 -> Data Type Conversion/1
  Data Type Conversion/1 -> Mux2/5
  S-R Flip-Flop/2 -> Data Type Conversion3/1
  Gen1 MCB Status/1 -> Logical Operator/1, Data Type Conversion1/1
  Bus Selector3/3 -> Compare To Zero3/1  "<Gen1_Open_MCB>"
  Bus Selector/2 -> Logical Operator2/2  "<Gen1_Fuel>"
  Bus Selector/1 -> Logical Operator2/1  "<Gen1_Starter>"
  Constant/1 -> Add1/1, Add/2
  Add1/1 -> Gen1 MCB/1
  Add/1 -> Gen1 GCB/1
  S-R Flip-Flop1/1 -> Add1/2
  Compare To Zero3/1 -> S-R Flip-Flop1/1
  Compare To Zero4/1 -> S-R Flip-Flop1/2
  Bus Selector3/4 -> Compare To Zero4/1  "<Gen1_Close_MCB>"
  Compare To Zero1/1 -> S-R Flip-Flop/2
  Compare To Zero/1 -> S-R Flip-Flop/1
  S-R Flip-Flop/1 -> Data Type Conversion2/1, Add/1
  Bus Creator/1 -> DIn1/1
  Din_Wood/1 -> Bus Selector/1, Bus Selector3/1
  Bus Selector3/1 -> Compare To Zero/1  "<Gen1_Open_GCB>"
  Bus Selector3/2 -> Compare To Zero1/1  "<Gen1_Close_GCB>"
  Data Type Conversion4/1 -> Gen1 Fuel Enable/1
  Constant1/1 -> Mux2/1  "Estop"

== system INTEGRATION_TEST_01/SS_Relays_and_Woodward/HWCtrl/Woodward Outputs - NGCHP - Gen1/DOUT type config ==
  note: The Constants are used to select Digital Output type:
      | - 0: Time-Stamped Digital Output
      | - 1: Pulse-Width Modulated DIgital Output
  DataIn Send : rtio_opalrt_common/DataIn Send  CtrlName='OpCtrl'  FcnNos=11  width=1  portType=double  checkVersion=off  expectedId=0  expectedVersion=0  opComp=>=
      settings: AttributesFormatString=%<CtrlName>
  DataIn Send1 : rtio_opalrt_common/DataIn Send  CtrlName='OpCtrl'  FcnNos=12  width=1  portType=double  checkVersion=off  expectedId=0  expectedVersion=0  opComp=>=
      settings: AttributesFormatString=%<CtrlName>
  Subsection 3 DOUT type : Constant
  Subsection 4 DOUT type : Constant
  Terminator1 : Terminator
  Terminator2 : Terminator
  wires:
  DataIn Send/1 -> Terminator2/1
  DataIn Send1/1 -> Terminator1/1
  Subsection 4 DOUT type/1 -> DataIn Send1/1
  Subsection 3 DOUT type/1 -> DataIn Send/1

== system INTEGRATION_TEST_01/SS_Relays_and_Woodward/HWCtrl/Woodward Outputs - NGCHP - Gen1/Woodward Primary Inputs - Gen1 ==
  note: Copyright (c) 2016 Massachusetts Institute of Technology
      | Permission is hereby granted, free of charge, to any person obtaining a copy of this software and associated documentation files (the "Software"), to deal
      | in the Software without restriction, including without limitation the rights to use, copy, modify, merge, publish, distribute, sublicense, and/or sell copies of the
      | Software, and to permit persons to whom the Software is furnished to do so, subject to the following conditions:
      |
      | THE SOFTWARE IS PROVIDED "AS IS", WITHOUT WARRANTY OF ANY KIND, EXPRESS OR IMPLIED, INCLUDING BUT NOT LIMITED TO THE
      | WARRANTIES OF MERCHANTABILITY, FITNESS FOR A PARTICULAR PURPOSE AND NONINFRINGEMENT. IN NO EVENT SHALL THE AUTHORS
      | OR COPYRIGHT HOLDERS BE LIABLE FOR ANY CLAIM, DAMAGES OR OTHER LIABILITY, WHETHER IN AN ACTION OF CONTRACT, TORT OR
      | OTHERWISE, ARISING FROM, OUT OF OR IN CONNECTION WITH THE SOFTWARE OR THE USE OR OTHER DEALINGS IN THE SOFTWARE
  note: NG-CHP -> Gen1
  WoodwardBias : Inport
  Bus Creator : BusCreator
  Bus Selector5 : BusSelector  OutputSignals=gen1_GOV_bias,gen1_AVR_bias
  Constant3 : Constant  Value=0
  Constant4 : Constant  Value=0
  Divide : Product  Inputs=*/
  Divide1 : Product  Inputs=*/
  Gen1 Ref AVR : Constant  Value=1.00
  Gen1 Ref GOV : Constant  Value=1.00
  Lowpass Filter : Subsystem  DialogController=fdesignblkfcn  DialogControllerArgs=DataTag2  InitFcn=fdesignblkfcn(gcbh, {'InitFcn'});  mask(Lowpass Filter){}
      mask help: Design a lowpass filter
      settings: CopyFcn=fdesignblkfcn(gcbh, {'CopyFcn'});
      mask Help: helpview(mapfilelocation('dsp'), 'dsplowpassfilter');
      mask Display: disp('Lowpass')
  Lowpass Filter1 : Subsystem  DialogController=fdesignblkfcn  DialogControllerArgs=DataTag4  InitFcn=fdesignblkfcn(gcbh, {'InitFcn'});  mask(Lowpass Filter){}
      mask help: Design a lowpass filter
      settings: CopyFcn=fdesignblkfcn(gcbh, {'CopyFcn'});
      mask Help: helpview(mapfilelocation('dsp'), 'dsplowpassfilter');
      mask Display: disp('Lowpass')
  ScalingBias : Constant  Value=20
  SimulatedBiasValues : Constant  Value=0
  Sum : Sum  Inputs=|+-
  Sum1 : Sum  Inputs=|+-
  Switch : Switch  Threshold=0.5
  Switch1 : Switch  Threshold=0.5
  bias_enable_for_woodward_ctrl : Constant
  Gen1 Gov and AVR : Outport
  wires:
  Bus Selector5/2 -> Divide1/1  "<gen1_AVR_bias>"
  Bus Selector5/1 -> Divide/1  "<gen1_GOV_bias>"
  WoodwardBias/1 -> Bus Selector5/1
  Bus Creator/1 -> Gen1 Gov and AVR/1
  Gen1 Ref GOV/1 -> Bus Creator/1  "Gen1 Ref GOV"
  Gen1 Ref AVR/1 -> Bus Creator/2  "Gen1 Ref AVR"
  Lowpass Filter1/1(Out) -> Switch1/1
  Lowpass Filter/1(Out) -> Switch/1
  bias_enable_for_woodward_ctrl/1 -> Switch/2, Switch1/2
  SimulatedBiasValues/1 -> Switch1/3, Switch/3
  Sum1/1 -> Lowpass Filter1/1(In)
  Switch1/1 -> Bus Creator/4  "Gen1 AVR"
  Switch/1 -> Bus Creator/3  "Gen1 Gov"
  Sum/1 -> Lowpass Filter/1(In)
  Constant4/1 -> Sum1/2
  Constant3/1 -> Sum/2
  Divide1/1 -> Sum1/1
  Divide/1 -> Sum/1
  ScalingBias/1 -> Divide1/2, Divide/2

== system INTEGRATION_TEST_01/SS_Relays_and_Woodward/UDP - Signal Formatting Block/MID-Checker/RMS ==
  s : Inport
  Discrete  Mean value6 : powerlib_extras/Discrete Measurements/Discrete  Mean value  Freq=60  Vinit=0  Ts=Ts
  Product3 : Product  RndMeth=Zero
  Signed Sqrt : Sqrt  SaturateOnIntegerOverflow=on
  S : Outport
  wires:
  s/1 -> Product3/1, Product3/2
  Product3/1 -> Discrete  Mean value6/1
  Discrete  Mean value6/1 -> Signed Sqrt/1
  Signed Sqrt/1 -> S/1

== system INTEGRATION_TEST_01/SS_Relays_and_Woodward/UDP - Signal Formatting Block/NG-Checker/RMS ==
  s : Inport
  Discrete  Mean value6 : powerlib_extras/Discrete Measurements/Discrete  Mean value  Freq=60  Vinit=0  Ts=Ts
  Product3 : Product  RndMeth=Zero
  Signed Sqrt : Sqrt  SaturateOnIntegerOverflow=on
  S : Outport
  wires:
  s/1 -> Product3/1, Product3/2
  Product3/1 -> Discrete  Mean value6/1
  Discrete  Mean value6/1 -> Signed Sqrt/1
  Signed Sqrt/1 -> S/1

== system INTEGRATION_TEST_01/SS_Relays_and_Woodward/UDP - Signal Formatting Block/UDP Data - Formatted Send - Integartion Test 1/Ethernet communication interface ==
  note: Ethernet communication interface example model
  Data trigger : Inport
  Data to send : Inport  Port=2
  AsyncEthernetCtrl : S-Function  InitFcn=generic_ethernet_cb('initfcn');  FunctionName=sfun_gen_async_ctrl  Parameters=ctrl_id, nbr_to_remote_endpoint, type_to_remote_endpoint,nbr_from_remote_endpoint,type_from_remote_endpoint,protocol,tcp_mode, port, offset_to_remote_endpoint,offset_from_remote_endpoint,swap_tx,swap_rx,0,nic_name,remote_ip,'','','','','','','','','','',exe_name,0  EnableBusSupport=off  mask(AsyncEthernetCtrl){ctrl_id=1, nbr_to_remote_endpoint=730, type_to_remote_endpoint=INT16, offset_to_remote_endpoint=0, nbr_from_remote_endpoint=4, type_from_remote_endpoint=UINT16, offset_from_remote_endpoint=0, nic_name=eth0, protocol=UDP, tcp_mode=Server, port=7200, remote_ip=255.255.255.255, exe_name=AsyncEthernet, swap_tx=off, swap_rx=off}
      mask prompts: ctrl_id "Controller ID"; nbr_to_remote_endpoint "Number of data to send"; type_to_remote_endpoint "Type of data to send"; offset_to_remote_endpoint "Byte offset of transmission buffer"; nbr_from_remote_endpoint "Number of data expected to be received"; type_from_remote_endpoint "Type of data expected to be received"; offset_from_remote_endpoint "Byte offset of reception buffer"; nic_name "Network interface name"; tcp_mode "TCP mode"; remote_ip "Remote IP address"; exe_name "Name of the executable"; swap_tx "Swap data endianness before transmission"; swap_rx "Swap data endianness after reception"
      mask help: Generic asynchronous process configuration block
      mask Help: eval('rtlab_help(''opasyncgenctrl'');');
      mask TypeOptions type_to_remote_endpoint: UINT8 | INT8 | UINT16 | INT16 | UINT32 | INT32 | FLOAT | DOUBLE
      mask TypeOptions type_from_remote_endpoint: UINT8 | INT8 | UINT16 | INT16 | UINT32 | INT32 | FLOAT | DOUBLE
      mask TypeOptions protocol: UDP | TCP
      mask TypeOptions tcp_mode: Client | Server
      mask Display: disp(sprintf('\nEthernet communication \ninterface controller\n'))
  B-width : SignalSpecification  Dimensions=nbr_from_remote_endpoint
  Constant : Constant  Value=1000
  Logo : opal_lib/Logo1  vide=[]
  Mux : Mux  Inputs=2
  OpAsyncRecv : rtlab/Communication/Asynchronous/OpAsyncRecv  ctl_id=ctrl_id  recv_id=ctrl_id  enable_param=off  fp1=1  fp2=2  fp3=3  fp4=4  fp5=5  sp1=string1  sp2=string2  sp3=string3  sp4=string4  sp5=string5
  OpAsyncSend : rtlab/Communication/Asynchronous/OpAsyncSend  ctl_id=ctrl_id  send_id=ctrl_id  mode=DONT_NEED_REPLY  enable_param=off  fp1=1  fp2=2  fp3=3  fp4=4  fp5=5  sp1=string1  sp2=string2  sp3=string3  sp4=string4  sp5=string5
  Terminator : Terminator
  Data received : Outport
  Status : Outport  Port=2
  wires:
  B-width/1 -> Data received/1
  OpAsyncRecv/3 -> B-width/1
  OpAsyncRecv/2 -> Terminator/1
  Constant/1 -> OpAsyncRecv/1
  Mux/1 -> Status/1
  OpAsyncRecv/1 -> Mux/2
  OpAsyncSend/1 -> Mux/1
  Data trigger/1 -> OpAsyncSend/1
  Data to send/1 -> OpAsyncSend/2

== system INTEGRATION_TEST_01/SS_Relays_and_Woodward/HWCtrl/Woodward Outputs - NGCHP - Gen1/DIO - Gr3/Conditioning ==
  In1 : Inport
  Bus Creator : BusCreator  Inputs=8
  Demux : Demux  Outputs=8
  Out1 : Outport
  wires:
  In1/1 -> Demux/1
  Bus Creator/1 -> Out1/1  "DI_CH00-07"
  Demux/8 -> Bus Creator/8  "Gen1_Alarm_CF"
  Demux/7 -> Bus Creator/7  "Gen1_Alarm_AB"
  Demux/6 -> Bus Creator/6  "Gen1_Open_MCB"
  Demux/5 -> Bus Creator/5  "Gen1_Close_MCB"
  Demux/4 -> Bus Creator/4  "Gen1_Open_GCB"
  Demux/3 -> Bus Creator/3  "Gen1_Close_GCB"
  Demux/2 -> Bus Creator/2  "Gen1_Fuel"
  Demux/1 -> Bus Creator/1  "Gen1_Starter"

== system INTEGRATION_TEST_01/SS_Relays_and_Woodward/HWCtrl/Woodward Outputs - NGCHP - Gen1/Woodward Primary Inputs - Gen1/Lowpass Filter ==
  In : Inport
  Generated Filter Block : DiscreteFir  Tag=BlockMethodSubSystem  Coefficients=[0.0069552863617617106 0.014587901014631248 -0.0057896483056441538 -0.056861876528372622 -0.059476680260783142 0.076118200884714562 0.29579154768342669 0.40638624201187618 0.29579154768342669 0.076118200884714562 -0.059476680260783142 -0.056861876528372622 -0.0057896483056441538 0.014587901014631248 0.0069552863617617106]  InputProcessing=Columns as channels (frame based)
  Out : Outport
  wires:
  Generated Filter Block/1 -> Out/1
  In/1 -> Generated Filter Block/1

== system INTEGRATION_TEST_01/SS_Relays_and_Woodward/HWCtrl/Woodward Outputs - NGCHP - Gen1/Woodward Primary Inputs - Gen1/Lowpass Filter1 ==
  In : Inport
  Generated Filter Block : DiscreteFir  Tag=BlockMethodSubSystem  Coefficients=[0.0069552863617617106 0.014587901014631248 -0.0057896483056441538 -0.056861876528372622 -0.059476680260783142 0.076118200884714562 0.29579154768342669 0.40638624201187618 0.29579154768342669 0.076118200884714562 -0.059476680260783142 -0.056861876528372622 -0.0057896483056441538 0.014587901014631248 0.0069552863617617106]  InputProcessing=Columns as channels (frame based)
  Out : Outport
  wires:
  Generated Filter Block/1 -> Out/1
  In/1 -> Generated Filter Block/1

== matlab function SS_Relays_and_Woodward/UDP - Signal Formatting Block/UDP Data - Formatted Send - Integartion Test 1/Cast uint16 ==
  data: u input double; y output double
function y = fcn(u)
%#codegen

x = double(typecast(uint32(u),'uint16'));
y = x(1); % low bits

== matlab function SS_Relays_and_Woodward/UDP - Signal Formatting Block/UDP Data - Formatted Send - Integartion Test 1/MATLAB Function ==
  data: u input double; y output double; sync output double
function [y, sync] = fcn(u)
%#codegen

[y, sync] = scopeBuffer(u);
